simulink model "q20c"  (R2016a)
settings: Solver=VariableStepAuto  StartTime=0.0  StopTime=10.0  RelTol=1e-3
settings Model: Creator=Satya  LastModifiedBy=Satya

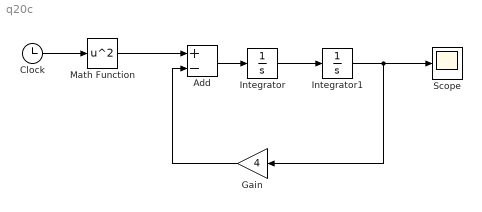
== system q20c ==
  Add : Sum  Inputs=+-
  Clock : Clock
  Gain : Gain  Gain=4
  Integrator : Integrator  InitialCondition=2
  Integrator1 : Integrator  InitialCondition=1
  Math Function : Math  Operator=square  SaturateOnIntegerOverflow=on
  Scope : Scope
  wires:
  Clock/1 -> Math Function/1
  Add/1 -> Integrator/1
  Integrator/1 -> Integrator1/1
  Math Function/1 -> Add/1
  Integrator1/1 -> Scope/1, Gain/1
  Gain/1 -> Add/2
